simulink library "Lib_Thermo_PT2S_TMATS_org"  (Simulink 10.0)
settings: Solver=ode45  StartTime=0.0  StopTime=10.0  RelTol=1e-3  EnableMultiTasking=on
Description:
  | Thomas Modules
settings Model: Creator=jwchapm2  LastModifiedBy=bhisma

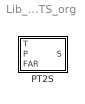
== system Lib_Thermo_PT2S_TMATS_org ==
  PT2S : Subsystem  mask(T-MATS: PT2S Library Block){}
      mask help: This block emperically calculates entropy (S) from pressure (P), temperature (T) and fuel to air ratio (FAR).
      mask Help: web(which('Thermo_TMATS_PT2S.html'),'-helpbrowser')

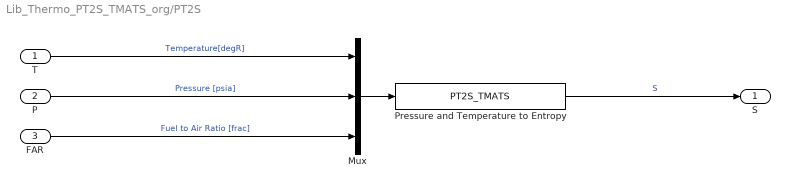
== system Lib_Thermo_PT2S_TMATS_org/PT2S ==
  T : Inport
  P : Inport  Port=2
  FAR : Inport  Port=3
  Mux : Mux  Inputs=3
  Pressure and Temperature to Entropy : S-Function  FunctionName=PT2S_TMATS  SFunctionModules='pt2sc_TMATS'  SFunctionDeploymentMode=off  EnableBusSupport=off
  S : Outport
  wires:
  Pressure and Temperature to Entropy/1 -> S/1  "S"
  Mux/1 -> Pressure and Temperature to Entropy/1
  T/1 -> Mux/1  "Temperature[degR]"
  FAR/1 -> Mux/3  "Fuel to Air Ratio [frac]"
  P/1 -> Mux/2  "Pressure [psia]"
